simulink model "MBD_FOC_SENSORLESS_MODEL"  (R2022b)
settings: Solver=FixedStepDiscrete  StartTime=0.0  StopTime=9  FixedStep=.00005  RelTol=1e-3  EnableMultiTasking=on
PostLoadFcn:
  | MBD_FOC_SENSORLESS_DATA;
InitFcn:
  | MBD_FOC_SENSORLESS_DATA;
model workspace (MAT data in the model file):
  mwTaskManagerKernelLatency = 1e-06
values from neighbouring files (symbols this model uses):
  Iq_Ref_openLoop = 0.5    [MBD_FOC_SENSORLESS_DATA.m]
  PI_params = mcb.internal.SetControllerParameters(pmsm,inverter,PU_System,T_pwm,Ts,Ts_speed)    [MBD_FOC_SENSORLESS_DATA.m]
  PU_System = mcb_SetPUSystem(pmsm,inverter)    [MBD_FOC_SENSORLESS_DATA.m]
  PWM1max = 1600    [MBD_FOC_SENSORLESS_DATA.m]
  PWM_frequency = 20e3    (= 20000)    [MBD_FOC_SENSORLESS_DATA.m]
  Speed_Ref_openLoop = 500    [MBD_FOC_SENSORLESS_DATA.m]
  Ts = T_pwm    (= 5e-05)    [MBD_FOC_SENSORLESS_DATA.m]
  Ts_speed = 30*Ts    (= 0.0015)    [MBD_FOC_SENSORLESS_DATA.m]
undefined symbols (not defined in the file or in its folder): DiscIntNeverNeededParam, inverter, pmsm
libraries: mcbcontrolslib x9, simulink x4, slpidlib x3, mcbplantlib x1, autolibpmsmexterior x1
(part 1 of 2)
settings Model: Creator=M91449  LastModifiedBy=Administrator
settings SolverCC: AlgebraicLoopSolver=TrustRegion  PositivePriorityOrder=on  AutoInsertRateTranBlk=on  InsertRTBMode=Always
settings DataIOCC: LimitDataPoints=on  ReturnWorkspaceOutputs=off
settings OptimizationCC: DefaultParameterBehavior=Inlined  PassReuseOutputArgsAs=Individual arguments  ZeroExternalMemoryAtStartup=off  ZeroInternalMemoryAtStartup=off  MaxStackSize=64  OptimizationLevel=level1  OptimizationCustomize=off  EfficientTunableParamExpr=on
settings DebuggingCC: MultiTaskDSMMsg=none  ParameterOverflowMsg=none  ParameterTunabilityLossMsg=error  UnconnectedInputMsg=warning  UnconnectedOutputMsg=warning  UnconnectedLineMsg=warning  SFUnexpectedBacktrackingDiag=warning  SFNoUnconditionalDefaultTransitionDiag=warning  SFExecutionAtInitializationDiag=none  SFMachineParentedDataDiag=warning  ArithmeticOperatorsInVariantConditions=warning
settings HardwareCC: ProdBitPerPointer=32  ProdBitPerSizeT=32  ProdBitPerPtrDiffT=32  ProdLargestAtomicInteger=Long  ProdLargestAtomicFloat=Double  ProdWordSize=32  ProdHWDeviceType=ARM Compatible->ARM Cortex-M  HardwareBoardFeatureSet=SoCBlockset
settings ModelReferenceCC: EnableRefExpFcnMdlSchedulingChecks=on  ModelReferenceNumInstancesAllowed=Single  PropagateSignalLabelsOutOfModel=off
settings SFSimCC: SimUseLocalCustomCode=off  MATLABDynamicMemAlloc=off  CustomCodeUndefinedFunction=UseInterfaceOnly
settings RTWCC: Description=Embedded Coder  SystemTargetFile=ert.tlc  GenCodeOnly=on  TemplateMakefile=ert_default_tmf  GenerateReport=on  RTWUseLocalCustomCode=off  IncludeHyperlinkInReport=on  LaunchReport=on  GenerateCodeMetricsReport=on  DLArmComputeVersion=19.05
settings CodeAppCC: ForceParamTrailComments=on  IgnoreCustomStorageClasses=off  MaxIdLength=255  OperatorAnnotations=on  SimulinkDataObjDesc=on  SFDataObjDesc=on  InsertBlockDesc=on
settings ERTTargetCC: GenerateSampleERTMain=on  InlinedParameterPlacement=NonHierarchical  ERTCustomFileTemplate=example_file_process.tlc
settings ConfigComp: CovMetricSettings=dw  CovSaveCumulativeToWorkspaceVar=on  CovSaveSingleToWorkspaceVar=on  CovExternalEMLEnable=off

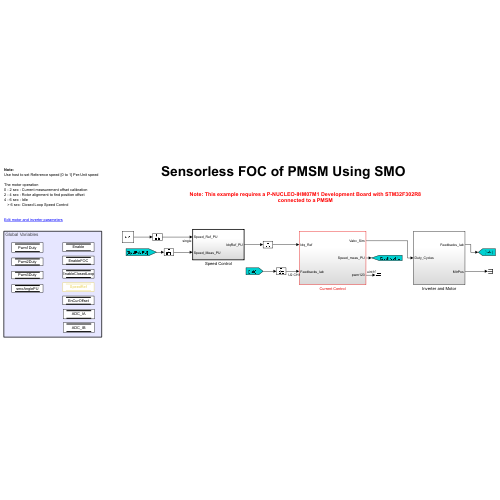
[thumbnail: Simulink's stored preview of the top-level diagram]
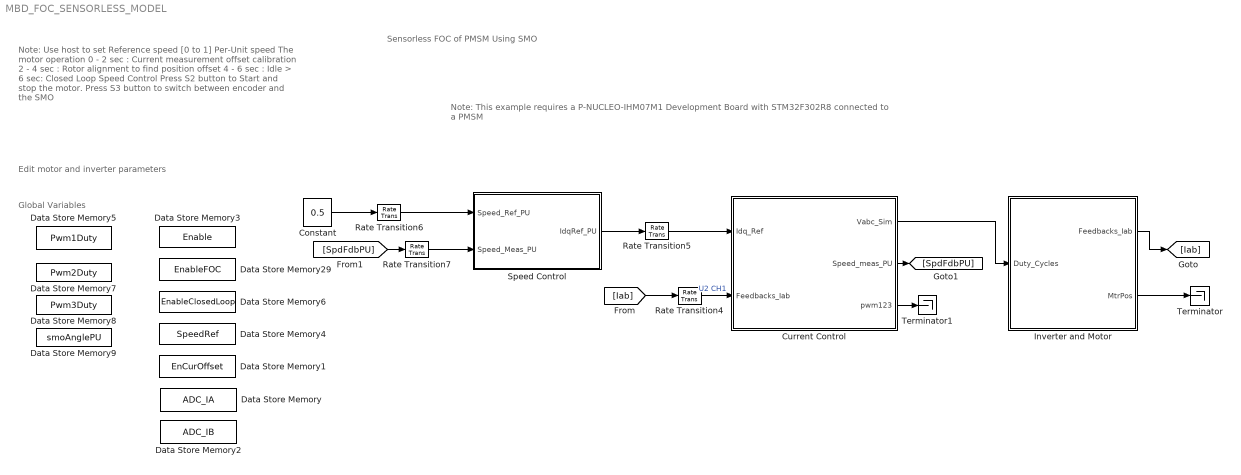
== system MBD_FOC_SENSORLESS_MODEL ==
  note: Edit motor and inverter parameters
  note: Note:
      | Use host to set Reference speed [0 to 1] Per-Unit speed
      |
      | The motor operation
      | 0 - 2 sec : Current measurement offset calibration
      | 2 - 4 sec : Rotor alignment to find position offset
      | 4 - 6 sec : Idle
      | > 6 sec: Closed Loop Speed Control
      |
      | Press S2 button to Start and stop the motor.
      | Press S3 button to switch between encoder and the SMO
  note: Global Variables
  note: Sensorless FOC of PMSM Using SMO
  note: Note: This example requires a P-NUCLEO-IHM07M1 Development Board with STM32F302R8 connected to a PMSM
  Constant : Constant  Value=0.5  OutDataTypeStr=single
  Current Control : Subsystem  VariantControl=Optimized
  Data Store Memory : DataStoreMemory  DataStoreName=ADC_IA  WriteAfterWriteMsg=warning  ShowAdditionalParam=off  OutDataTypeStr=uint16
  Data Store Memory1 : DataStoreMemory  DataStoreName=EnCurOffset  ShowAdditionalParam=off  OutDataTypeStr=boolean
  Data Store Memory2 : DataStoreMemory  DataStoreName=ADC_IB  WriteAfterWriteMsg=warning  ShowAdditionalParam=off  OutDataTypeStr=uint16
  Data Store Memory29 : DataStoreMemory  DataStoreName=EnableFOC  ShowAdditionalParam=off  OutDataTypeStr=boolean
  Data Store Memory3 : DataStoreMemory  DataStoreName=Enable  ShowAdditionalParam=off  OutDataTypeStr=boolean
  Data Store Memory4 : DataStoreMemory  DataStoreName=SpeedRef  ShowAdditionalParam=off  OutDataTypeStr=dataType
  Data Store Memory5 : DataStoreMemory  DataStoreName=Pwm1Duty  WriteAfterWriteMsg=warning  ShowAdditionalParam=off  OutDataTypeStr=uint16
  Data Store Memory6 : DataStoreMemory  DataStoreName=EnableClosedLoop  ShowAdditionalParam=off  OutDataTypeStr=boolean
  Data Store Memory7 : DataStoreMemory  DataStoreName=Pwm2Duty  WriteAfterWriteMsg=warning  ShowAdditionalParam=off  OutDataTypeStr=uint16
  Data Store Memory8 : DataStoreMemory  DataStoreName=Pwm3Duty  WriteAfterWriteMsg=warning  ShowAdditionalParam=off  OutDataTypeStr=uint16
  Data Store Memory9 : DataStoreMemory  DataStoreName=smoAnglePU  WriteAfterWriteMsg=warning  ShowAdditionalParam=off  OutDataTypeStr=dataType
  Inverter and Motor : Subsystem
  Rate Transition{4..7} (4 alike) : RateTransition  Deterministic=off
  Speed Control : Subsystem  TreatAsAtomicUnit=on  SystemSampleTime=Ts_speed
  Terminator : Terminator
  Terminator1 : Terminator
  wires:
  Current Control/1(Vabc_Sim) -> Inverter and Motor/1(Duty_Cycles)
  Rate Transition4/1 -> Current Control/2(Feedbacks_Iab)  "U2 CH1"
  Rate Transition6/1 -> Speed Control/1(Speed_Ref_PU)
  Rate Transition7/1 -> Speed Control/2(Speed_Meas_PU)
  Speed Control/1(IdqRef_PU) -> Rate Transition5/1
  Inverter and Motor/1(Feedbacks_Iab) -> [Iab]
  [Iab] -> Rate Transition4/1
  Rate Transition5/1 -> Current Control/1(Idq_Ref)
  Constant/1 -> Rate Transition6/1
  Inverter and Motor/2(MtrPos) -> Terminator/1
  Current Control/3(pwm123) -> Terminator1/1
  [SpdFdbPU] -> Rate Transition7/1
  Current Control/2(Speed_meas_PU) -> [SpdFdbPU]

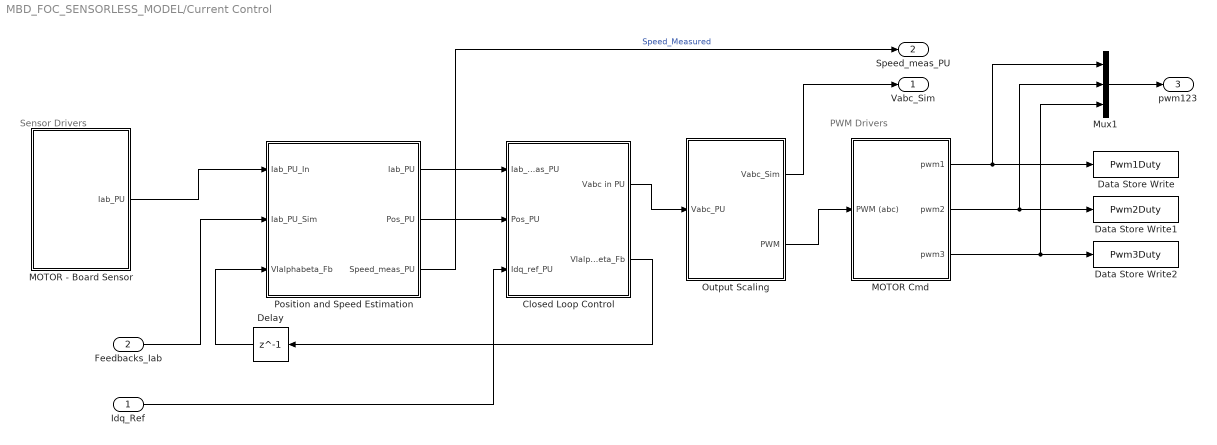
== system MBD_FOC_SENSORLESS_MODEL/Current Control ==
  note: Sensor Drivers
  note: PWM Drivers
  Idq_Ref : Inport
  Feedbacks_Iab : Inport  Port=2
  Closed Loop Control : Subsystem
  Data Store Write : DataStoreWrite  DataStoreName=Pwm1Duty  DataStoreElements=Pwm1Duty  IndexOptions=Index vector (dialog)  Indices=1  OutputSizes=1
  Data Store Write1 : DataStoreWrite  DataStoreName=Pwm2Duty  DataStoreElements=Pwm2Duty  IndexOptions=Index vector (dialog)  Indices=1  OutputSizes=1
  Data Store Write2 : DataStoreWrite  DataStoreName=Pwm3Duty  DataStoreElements=Pwm3Duty  IndexOptions=Index vector (dialog)  Indices=1  OutputSizes=1
  Delay : Delay  DelayLength=1
  MOTOR Cmd : Subsystem
  MOTOR - Board Sensor : Subsystem
  Mux1 : Mux  Inputs=3
  Output Scaling : Subsystem
  Position and Speed Estimation : Subsystem
  Vabc_Sim : Outport
  Speed_meas_PU : Outport  Port=2
  pwm123 : Outport  Port=3  OutDataTypeStr=uint16
  wires:
  Closed Loop Control/1(Vabc in PU) -> Output Scaling/1(Vabc_PU)
  Output Scaling/2(PWM) -> MOTOR Cmd/1(PWM (abc))
  Output Scaling/1(Vabc_Sim) -> Vabc_Sim/1
  Feedbacks_Iab/1 -> Position and Speed Estimation/2(Iab_PU_Sim)
  Position and Speed Estimation/1(Iab_PU) -> Closed Loop Control/1(Iab_meas_PU)
  Position and Speed Estimation/2(Pos_PU) -> Closed Loop Control/2(Pos_PU)
  MOTOR - Board Sensor/1(Iab_PU) -> Position and Speed Estimation/1(Iab_PU_In)
  Idq_Ref/1 -> Closed Loop Control/3(Idq_ref_PU)
  Closed Loop Control/2(VIalphabeta_Fb) -> Delay/1
  Delay/1 -> Position and Speed Estimation/3(VIalphabeta_Fb)
  Position and Speed Estimation/3(Speed_meas_PU) -> Speed_meas_PU/1  "Speed_Measured"
  MOTOR Cmd/3(pwm3) -> Mux1/3, Data Store Write2/1
  MOTOR Cmd/1(pwm1) -> Mux1/1, Data Store Write/1
  MOTOR Cmd/2(pwm2) -> Mux1/2, Data Store Write1/1
  Mux1/1 -> pwm123/1

== system MBD_FOC_SENSORLESS_MODEL/Inverter and Motor ==
  Duty_Cycles : Inport
  Codegeneration : Subsystem
  Simulation : Subsystem
  Variant Sink : VariantSink
  Variant Source : VariantSource
  Feedbacks_Iab : Outport  VectorParamsAs1DForOutWhenUnconnected=off
  MtrPos : Outport  Port=2
  wires:
  Codegeneration/1(Feedbacks_Iab) -> Variant Source/1
  Variant Sink/1 -> Codegeneration/1(Duty_Cycles)
  Simulation/1(Feedbacks_Iab) -> Variant Source/2
  Variant Sink/2 -> Simulation/1(Duty_Cycles)
  Variant Source/1 -> Feedbacks_Iab/1
  Duty_Cycles/1 -> Variant Sink/1
  Simulation/2(MtrPos) -> MtrPos/1

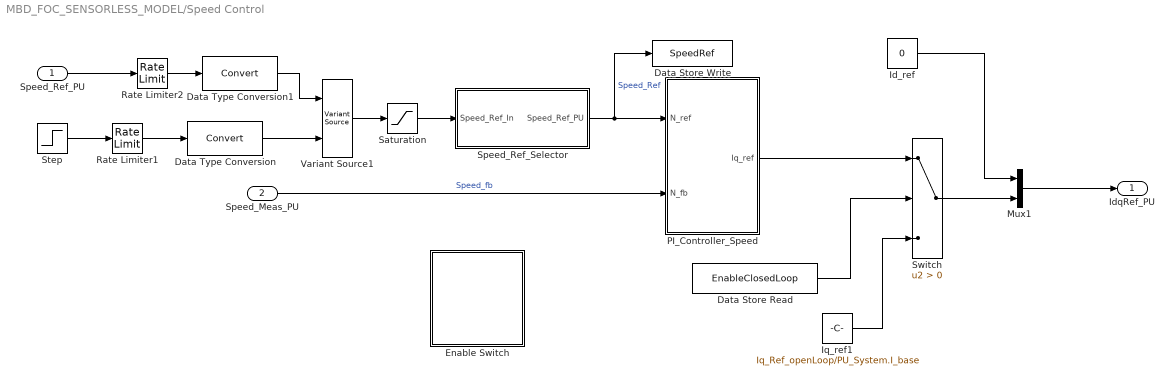
== system MBD_FOC_SENSORLESS_MODEL/Speed Control ==
  Speed_Ref_PU : Inport  OutDataTypeStr=single
  Speed_Meas_PU : Inport  Port=2
  Data Store Read : DataStoreRead  DataStoreName=EnableClosedLoop  IndexOptions=Index vector (dialog)  Indices=1  OutputSizes=1
  Data Store Write : DataStoreWrite  DataStoreName=SpeedRef  IndexOptions=Index vector (dialog)  Indices=1  OutputSizes=1
  Data Type Conversion : DataTypeConversion  SaturateOnIntegerOverflow=off  RndMeth=Floor
  Data Type Conversion1 : DataTypeConversion  SaturateOnIntegerOverflow=off  RndMeth=Floor
  Enable Switch : Subsystem  Variant=on  VariantControlMode=sim codegen switching
  Id_ref : Constant  Value=0  OutDataTypeStr=dataType  SampleTime=Ts_speed
  Iq_ref1 : Constant  Value=Iq_Ref_openLoop/PU_System.I_base  OutDataTypeStr=dataType  SampleTime=Ts_speed
  Mux1 : Mux  Inputs=2
  PI_Controller_Speed : Subsystem
  Rate Limiter1 : RateLimiter  RisingSlewLimit=0.5  FallingSlewLimit=-0.2  SampleTimeMode=inherited
  Rate Limiter2 : RateLimiter  RisingSlewLimit=0.5  FallingSlewLimit=-0.2  SampleTimeMode=inherited
  Saturation : Saturate  UpperLimit=(pmsm.N_max/PU_System.N_base)  LowerLimit=Speed_Ref_openLoop/PU_System.N_base
  Speed_Ref_Selector : Subsystem
  Step : Step  Time=5.5  Before=Speed_Ref_openLoop/PU_System.N_base  After=1.31  OutDataTypeStr=single
  Switch : Switch  Criteria=u2 > Threshold  SaturateOnIntegerOverflow=off  InputSameDT=off
  Variant Source1 : VariantSource
  IdqRef_PU : Outport  VectorParamsAs1DForOutWhenUnconnected=off
  wires:
  Speed_Meas_PU/1 -> PI_Controller_Speed/2(N_fb)  "Speed_fb"
  Id_ref/1 -> Mux1/1
  Mux1/1 -> IdqRef_PU/1
  Speed_Ref_Selector/1(Speed_Ref_PU) -> Data Store Write/1, PI_Controller_Speed/1(N_ref)  "Speed_Ref"
  Data Type Conversion/1 -> Variant Source1/2
  Step/1 -> Rate Limiter1/1
  Rate Limiter1/1 -> Data Type Conversion/1
  PI_Controller_Speed/1(Iq_ref) -> Switch/1
  Switch/1 -> Mux1/2
  Iq_ref1/1 -> Switch/3
  Data Store Read/1 -> Switch/2
  Variant Source1/1 -> Saturation/1
  Saturation/1 -> Speed_Ref_Selector/1(Speed_Ref_In)
  Speed_Ref_PU/1 -> Rate Limiter2/1
  Data Type Conversion1/1 -> Variant Source1/1
  Rate Limiter2/1 -> Data Type Conversion1/1

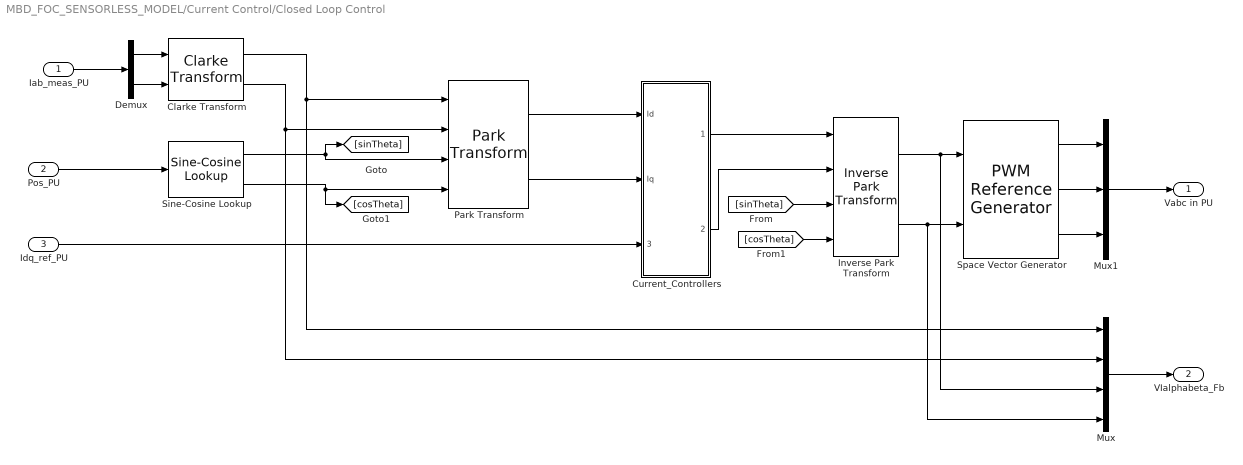
== system MBD_FOC_SENSORLESS_MODEL/Current Control/Closed Loop Control ==
  Iab_meas_PU : Inport
  Pos_PU : Inport  Port=2
  Idq_ref_PU : Inport  Port=3
  Clarke Transform : mcbcontrolslib/Clarke Transform  VariantControl=Variant2
  Current_Controllers : Subsystem
  Demux : Demux  Outputs=2
  Inverse Park Transform : mcbcontrolslib/Inverse Park Transform  AxisAlignment=D-axis
  Mux : Mux
  Mux1 : Mux  Inputs=3
  Park Transform : mcbcontrolslib/Park Transform  AxisAlignment=D-axis
  Sine-Cosine Lookup : mcbcontrolslib/Sine-Cosine Lookup  AngleInput=Per-unit  N_points=1024
  Space Vector Generator : mcbcontrolslib/PWM Reference Generator  inSignal=Valphabeta  modType=SVM: space vector modulation
  Vabc in PU : Outport  VectorParamsAs1DForOutWhenUnconnected=off
  VIalphabeta_Fb : Outport  Port=2
  wires:
  Current_Controllers/1(Vd_ref) -> Inverse Park Transform/1
  Inverse Park Transform/1 -> Mux/3, Space Vector Generator/1
  Park Transform/1 -> Current_Controllers/1(Id)
  Clarke Transform/1 -> Mux/1, Park Transform/1
  [sinTheta] -> Inverse Park Transform/3
  Sine-Cosine Lookup/1 -> Park Transform/3, [sinTheta]
  Clarke Transform/2 -> Mux/2, Park Transform/2
  Space Vector Generator/1 -> Mux1/1
  Space Vector Generator/3 -> Mux1/3
  Sine-Cosine Lookup/2 -> [cosTheta], Park Transform/4
  Space Vector Generator/2 -> Mux1/2
  Idq_ref_PU/1 -> Current_Controllers/3(Idq_ref_PU)
  Iab_meas_PU/1 -> Demux/1
  Inverse Park Transform/2 -> Mux/4, Space Vector Generator/2
  Demux/1 -> Clarke Transform/1
  Demux/2 -> Clarke Transform/2
  Park Transform/2 -> Current_Controllers/2(Iq)
  [cosTheta] -> Inverse Park Transform/4
  Current_Controllers/2(Vq_ref) -> Inverse Park Transform/2
  Mux1/1 -> Vabc in PU/1
  Pos_PU/1 -> Sine-Cosine Lookup/1
  Mux/1 -> VIalphabeta_Fb/1

== system MBD_FOC_SENSORLESS_MODEL/Current Control/MOTOR Cmd ==
  PWM (abc) : Inport
  Dead time Compensation : Bias  Bias=round( (inverter.deadtime/5e-5) *PWM1max )  SaturateOnIntegerOverflow=off
  Demux : Demux  Outputs=3
  Saturation low side turn on : Saturate  UpperLimit=PWM1max  LowerLimit=round( (inverter.deadtime/5e-5) *PWM1max )* 2
  int to uint : DataTypeConversion  OutDataTypeStr=uint16  ConvertRealWorld=Stored Integer (SI)  SaturateOnIntegerOverflow=off  RndMeth=Floor
  pwm1 : Outport  OutDataTypeStr=uint16
  pwm2 : Outport  Port=2  OutDataTypeStr=uint16
  pwm3 : Outport  Port=3  OutDataTypeStr=uint16
  wires:
  int to uint/1 -> Saturation low side turn on/1
  Dead time Compensation/1 -> int to uint/1
  PWM (abc)/1 -> Dead time Compensation/1
  Saturation low side turn on/1 -> Demux/1
  Demux/1 -> pwm1/1
  Demux/2 -> pwm2/1
  Demux/3 -> pwm3/1

== system MBD_FOC_SENSORLESS_MODEL/Current Control/MOTOR - Board Sensor ==
  Add2 : Sum  Inputs=+-  OutDataTypeStr=int16  RndMeth=Simplest
  Data Store Read : DataStoreRead  DataStoreName=EnCurOffset  IndexOptions=Index vector (dialog)  Indices=1  OutputSizes=1
  Data Store Read1 : DataStoreRead  DataStoreName=ADC_IA  IndexOptions=Index vector (dialog)  Indices=1  OutputSizes=1
  Data Store Read2 : DataStoreRead  DataStoreName=ADC_IB  IndexOptions=Index vector (dialog)  Indices=1  OutputSizes=1
  Mux2 : Mux  Inputs=2
  Offset1 : Subsystem
  Scale Ia Ib to (A) : DataTypeConversion  OutDataTypeStr=fixdt(1,16, 1.65/2048 / (inverter.Rshunt * inverter.opamp_Gain),0)  ConvertRealWorld=Stored Integer (SI)  SaturateOnIntegerOverflow=off  RndMeth=Floor
  To Per-Unit : Gain  Gain=inverter.invertingAmp/PU_System.I_base  OutMin=-1  OutMax=1  OutDataTypeStr=dataType  RndMeth=Zero
  Iab_PU : Outport  OutDataTypeStr=dataType  VectorParamsAs1DForOutWhenUnconnected=off
  wires:
  Mux2/1 -> Add2/1, Offset1/1(Iab)
  Scale Ia Ib to (A)/1 -> To Per-Unit/1  "Ia Ib"
  Offset1/1(Offset) -> Add2/2
  Add2/1 -> Scale Ia Ib to (A)/1
  Data Store Read/1 -> Offset1/Enable
  To Per-Unit/1 -> Iab_PU/1
  Data Store Read1/1 -> Mux2/1
  Data Store Read2/1 -> Mux2/2

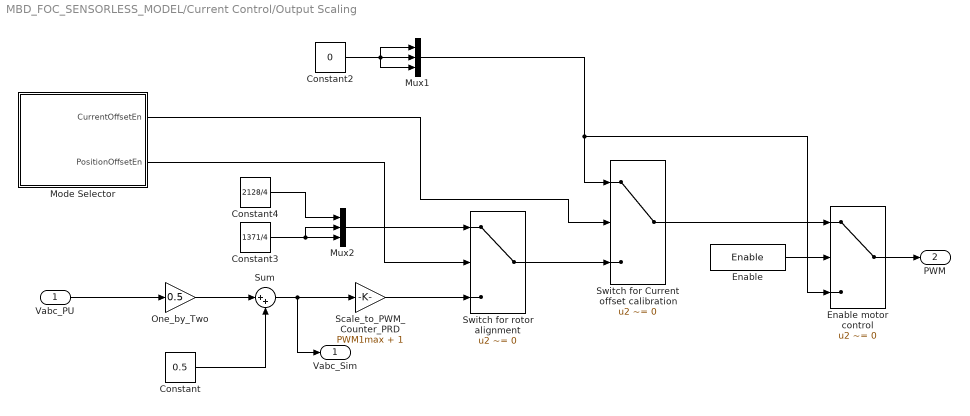
== system MBD_FOC_SENSORLESS_MODEL/Current Control/Output Scaling ==
  Vabc_PU : Inport
  Constant : Constant  Value=0.5  OutDataTypeStr=dataType  SampleTime=-1
  Constant2 : Constant  Value=0  OutDataTypeStr=Inherit: Inherit via back propagation
  Constant3 : Constant  Value=1371/4  OutDataTypeStr=Inherit: Inherit via back propagation
  Constant4 : Constant  Value=2128/4  OutDataTypeStr=Inherit: Inherit via back propagation
  Enable : DataStoreRead  DataStoreName=Enable  IndexOptions=Index vector (dialog)  Indices=1  OutputSizes=1
  Enable motor control : Switch  Criteria=u2 ~= 0  Threshold=250  SaturateOnIntegerOverflow=off  InputSameDT=off
  Mode Selector : Subsystem
  Mux1 : Mux  Inputs=3
  Mux2 : Mux  Inputs=3
  One_by_Two : Gain  Gain=0.5  RndMeth=Simplest  OutDataTypeStr=Inherit: Same as input
  Scale_to_PWM_Counter_PRD : Gain  Gain=PWM1max + 1  OutDataTypeStr=uint16  RndMeth=Simplest
  Sum : Sum  Inputs=|++
  Switch for Current offset calibration : Switch  Criteria=u2 ~= 0  Threshold=250  SaturateOnIntegerOverflow=off  InputSameDT=off
  Switch for rotor alignment : Switch  Criteria=u2 ~= 0  Threshold=250  SaturateOnIntegerOverflow=off  InputSameDT=off
  Vabc_Sim : Outport
  PWM : Outport  Port=2
  wires:
  Sum/1 -> Scale_to_PWM_Counter_PRD/1, Vabc_Sim/1
  Constant/1 -> Sum/2
  One_by_Two/1 -> Sum/1
  Switch for rotor alignment/1 -> Switch for Current offset calibration/3
  Vabc_PU/1 -> One_by_Two/1
  Mux2/1 -> Switch for rotor alignment/1
  Mux1/1 -> Switch for Current offset calibration/1, Enable motor control/3
  Constant2/1 -> Mux1/1, Mux1/3, Mux1/2
  Constant3/1 -> Mux2/3, Mux2/2
  Constant4/1 -> Mux2/1
  Enable/1 -> Enable motor control/2
  Mode Selector/2(PositionOffsetEn) -> Switch for rotor alignment/2
  Scale_to_PWM_Counter_PRD/1 -> Switch for rotor alignment/3
  Mode Selector/1(CurrentOffsetEn) -> Switch for Current offset calibration/2
  Enable motor control/1 -> PWM/1
  Switch for Current offset calibration/1 -> Enable motor control/1

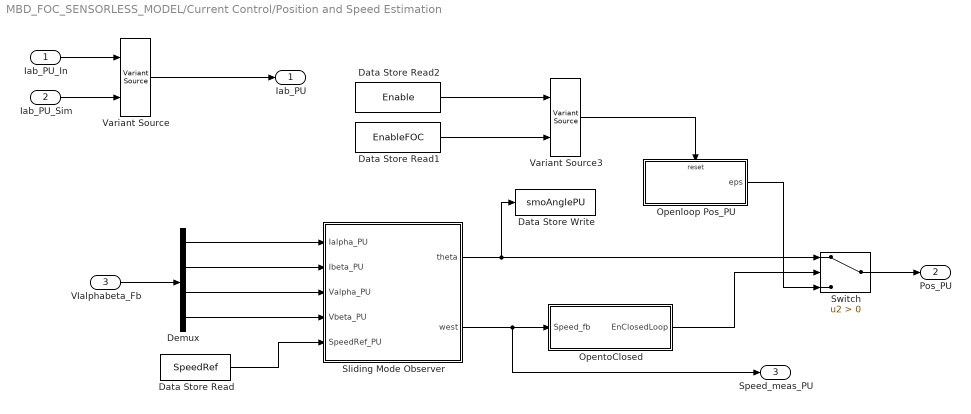
== system MBD_FOC_SENSORLESS_MODEL/Current Control/Position and Speed Estimation ==
  Iab_PU_In : Inport
  Iab_PU_Sim : Inport  Port=2
  VIalphabeta_Fb : Inport  Port=3
  Data Store Read : DataStoreRead  DataStoreName=SpeedRef  IndexOptions=Index vector (dialog)  Indices=1  OutputSizes=1
  Data Store Read1 : DataStoreRead  DataStoreName=EnableFOC  IndexOptions=Index vector (dialog)  Indices=1  OutputSizes=1
  Data Store Read2 : DataStoreRead  DataStoreName=Enable  IndexOptions=Index vector (dialog)  Indices=1  OutputSizes=1
  Data Store Write : DataStoreWrite  DataStoreName=smoAnglePU  IndexOptions=Index vector (dialog)  Indices=1  OutputSizes=1
  Demux : Demux
  Openloop Pos_PU : Subsystem  TreatAsAtomicUnit=on
  OpentoClosed : Subsystem
  Sliding Mode Observer : Subsystem
  Switch : Switch  Criteria=u2 > Threshold  SaturateOnIntegerOverflow=off  InputSameDT=off
  Variant Source : VariantSource
  Variant Source3 : VariantSource
  Iab_PU : Outport
  Pos_PU : Outport  Port=2
  Speed_meas_PU : Outport  Port=3
  wires:
  Iab_PU_In/1 -> Variant Source/1
  Iab_PU_Sim/1 -> Variant Source/2
  Variant Source/1 -> Iab_PU/1
  Data Store Read1/1 -> Variant Source3/2
  Variant Source3/1 -> Openloop Pos_PU/Reset
  Data Store Read2/1 -> Variant Source3/1
  VIalphabeta_Fb/1 -> Demux/1
  Demux/4 -> Sliding Mode Observer/4(Vbeta_PU)
  Data Store Read/1 -> Sliding Mode Observer/5(SpeedRef_PU)
  Demux/2 -> Sliding Mode Observer/2(Ibeta_PU)
  Demux/1 -> Sliding Mode Observer/1(Ialpha_PU)
  Demux/3 -> Sliding Mode Observer/3(Valpha_PU)
  Sliding Mode Observer/2(west) -> Speed_meas_PU/1, OpentoClosed/1(Speed_fb)
  OpentoClosed/1(EnClosedLoop) -> Switch/2
  Sliding Mode Observer/1(theta) -> Data Store Write/1, Switch/1
  Switch/1 -> Pos_PU/1
  Openloop Pos_PU/1(eps) -> Switch/3

== system MBD_FOC_SENSORLESS_MODEL/Inverter and Motor/Codegeneration ==
  Duty_Cycles : Inport
  Ground : Ground
  Terminator : Terminator
  Feedbacks_Iab : Outport  VectorParamsAs1DForOutWhenUnconnected=off
  wires:
  Ground/1 -> Feedbacks_Iab/1
  Duty_Cycles/1 -> Terminator/1

== system MBD_FOC_SENSORLESS_MODEL/Inverter and Motor/Simulation ==
  Duty_Cycles : Inport
  Bus Selector : BusSelector  OutputSignals=MtrPos
  Inverter : Subsystem
  Load_Profile (Torque) : Subsystem
  Sensor_Measurements : Subsystem
  Surface Mount PMSM : autolibpmsmexterior/Surface Mount PMSM  port_config=Torque  sim_type=Discrete  Ts=Ts  P=pmsm.p  Rs=pmsm.Rs + inverter.R_board  Ldq_=pmsm.Ld  KConstText=Permanent flux linkage constant (lambda_pm):  lambda_pm=pmsm.FluxPM  Ke=159.9771  Kt=1.323  mechanical=[pmsm.J, pmsm.B, 0]  idq0=[0 0]  theta_init=0  omega_init=0  KConst=pmsm.FluxPM  lambda_pm_calc=pmsm.FluxPM  RefBlkName='autolibpmsmexterior/Surface Mount PMSM'  aMode=5  Ldq="[0.0002      0.0002]"
  Terminator : Terminator
  Feedbacks_Iab : Outport  VectorParamsAs1DForOutWhenUnconnected=off
  MtrPos : Outport  Port=2
  wires:
  Duty_Cycles/1 -> Inverter/1(Duty_abc)
  Surface Mount PMSM/2 -> Sensor_Measurements/1(PhaseCurr)  "Iabc"
  Sensor_Measurements/1(Iab_fb) -> Feedbacks_Iab/1
  Load_Profile (Torque)/1(Load_Trq) -> Surface Mount PMSM/1
  Inverter/1(Vabc) -> Surface Mount PMSM/2
  Surface Mount PMSM/3 -> Terminator/1
  Surface Mount PMSM/1 -> Bus Selector/1
  Bus Selector/1 -> MtrPos/1  "<MtrPos>"

== system MBD_FOC_SENSORLESS_MODEL/Speed Control/Enable Switch ==
  Codegen : Subsystem  VariantControl=(codegen)
  Sim : Subsystem  VariantControl=(sim)

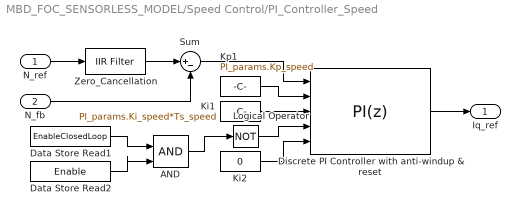
== system MBD_FOC_SENSORLESS_MODEL/Speed Control/PI_Controller_Speed ==
  N_ref : Inport
  N_fb : Inport  Port=2
  AND : Logic  IconShape=distinctive  AllPortsSameDT=off  OutDataTypeStr=boolean
  Data Store Read1 : DataStoreRead  DataStoreName=EnableClosedLoop  IndexOptions=Index vector (dialog)  Indices=1  OutputSizes=1
  Data Store Read2 : DataStoreRead  DataStoreName=Enable  IndexOptions=Index vector (dialog)  Indices=1  OutputSizes=1
  Discrete PI Controller with anti-windup & reset : slpidlib/PID Controller  Controller=PI  Form=Parallel  TimeDomain=Discrete-time  UseExternalTs=off  SampleTime=-1  IntegratorMethod=Forward Euler  FilterMethod=Forward Euler  ControllerParametersSource=external  P=1  I=1  UseKiTs=on  D=0  N=100  UseFilter=on  TunerSelectOption=Transfer Function Based (PID Tuner App)  InitialConditionSource=external  InitialConditionForIntegrator=0  InitialConditionForFilter=0  DifferentiatorICPrevScaledInput=0  ExternalReset=level  TrackingMode=off  Kt=1  LimitOutput=on  SatLimitsSource=internal  UpperSaturationLimit=1  LowerSaturationLimit=-1  LinearizeAsGain=on  AntiWindupMode=clamping  Kb=1  LimitIntegrator=off  UpperIntegratorSaturationLimit=inf  LowerIntegratorSaturationLimit=-inf  RndMeth=Simplest  POutMin=[]  POutMax=[]  IOutMin=[]  IOutMax=[]  DOutMin=[]  DOutMax=[]  NOutMin=[]  NOutMax=[]  SumOutMin=[]  SumOutMax=[]  SaturationOutDataTypeStr=Inherit: Inherit via back propagation  SaturationOutMin=[]  SaturationOutMax=[]  PParamMin=[]  PParamMax=[]  IParamMin=[]  IParamMax=[]  DParamMin=[]  DParamMax=[]  NParamMin=[]  NParamMax=[]  KbParamMin=[]  KbParamMax=[]  KtParamMin=[]  KtParamMax=[]  KbOutMin=[]  KbOutMax=[]  KtOutMin=[]  KtOutMax=[]  IntegratorOutMin=[]  IntegratorOutMax=[]  FilterOutMin=[]  FilterOutMax=[]  SumI1OutMin=[]  SumI1OutMax=[]  SumI2OutMin=[]  SumI2OutMax=[]  SumI3OutMin=[]  SumI3OutMax=[]  SumI4OutMin=[]  SumI4OutMax=[]  SumDOutMin=[]  SumDOutMax=[]  DifferentiatorOutMin=[]  DifferentiatorOutMax=[]  FilterDiffOutCoefMin=[]  FilterDiffOutCoefMax=[]  ReciprocalOutMin=[]  ReciprocalOutMax=[]  SumDenOutMin=[]  SumDenOutMax=[]  SumNumOutMin=[]  SumNumOutMax=[]  DivideOutMin=[]  DivideOutMax=[]  UdiffTsProdOutMin=[]  UdiffTsProdOutMax=[]  NTsProdOutMin=[]  NTsProdOutMax=[]  UintegralTsProdOutMin=[]  UintegralTsProdOutMax=[]  UngainTsProdOutMin=[]  UngainTsProdOutMax=[]  ClampingZeroOutDataTypeStr=Inherit: Inherit via back propagation  ClampingZeroOutMin=[]  ClampingZeroOutMax=[]  FilterDenConstantOutDataTypeStr=Inherit: Inherit via back propagation  FilterDenConstantOutMin=[]  FilterDenConstantOutMax=[]  PCopyOutDataTypeStr=Inherit: Inherit via back propagation  PCopyOutMin=[]  PCopyOutMax=[]  NCopyOutDataTypeStr=Inherit: Inherit via back propagation  NCopyOutMin=[]  NCopyOutMax=[]  IntegratorContinuousStateAttributes=''  IntegratorStateMustResolveToSignalObject=off  IntegratorRTWStateStorageClass=Auto  FilterContinuousStateAttributes=''  FilterStateMustResolveToSignalObject=off  FilterRTWStateStorageClass=Auto  ParallelPVariant=ExternalParameters  IdealPVariant=Disabled  IVariant=ExternalParameters  DVariant=Disabled  IntegratorVariant=Discrete  SatVariant=Enabled  AWVariant=DiscClampingParallel  PCopyVariant=Disabled  TRVariant=Disabled  FdbkBlocksVariant=Forward  IdealPFdbkVariant=Disabled  SatFdbkVariant=Disabled  DerivativeFilterVariant=Disabled  NVariant=Disabled  NCopyVariant=Disabled_SignalSpec  FilterICVariant=Disabled  IntegratorICVariant=ExternalICs  ExternalResetVariant=ExternalReset  TRSumVariant=Passthrough  SumFdbkVariant=Disabled  SumVariant=Sum_PI  TsampFilterVariant=InternalTs  TsampNgainVariant=Passthrough  TsampIntegralVariant=Passthrough  ExternalSaturationOutDataTypeStr=Inherit: Same as second input
  Ki1 : Constant  Value=PI_params.Ki_speed*Ts_speed  OutDataTypeStr=dataType  SampleTime=-1
  Ki2 : Constant  Value=0  OutDataTypeStr=dataType  SampleTime=-1
  Kp1 : Constant  Value=PI_params.Kp_speed  OutDataTypeStr=dataType  SampleTime=-1
  Logical Operator : Logic  Operator=NOT  IconShape=distinctive  AllPortsSameDT=off  OutDataTypeStr=boolean
  Sum : Sum  Inputs=|+-  OutDataTypeStr=Inherit: Same as first input
  Zero_Cancellation : mcbcontrolslib/IIR Filter  VariantControl=Low Pass Filter  VariantSelect=Low-pass  Filter_constant=0.001*(Ts_speed/Ts)  advancedSettings=off  Ts=50e-6  cutOff_freq=98.4464
  Iq_ref : Outport  VectorParamsAs1DForOutWhenUnconnected=off
  wires:
  Discrete PI Controller with anti-windup & reset/1 -> Iq_ref/1
  Ki1/1 -> Discrete PI Controller with anti-windup & reset/3
  Kp1/1 -> Discrete PI Controller with anti-windup & reset/2
  N_fb/1 -> Sum/2
  N_ref/1 -> Zero_Cancellation/1
  Sum/1 -> Discrete PI Controller with anti-windup & reset/1
  Logical Operator/1 -> Discrete PI Controller with anti-windup & reset/4
  Ki2/1 -> Discrete PI Controller with anti-windup & reset/5
  Zero_Cancellation/1 -> Sum/1
  AND/1 -> Logical Operator/1
  Data Store Read1/1 -> AND/1
  Data Store Read2/1 -> AND/2

== system MBD_FOC_SENSORLESS_MODEL/Speed Control/Speed_Ref_Selector ==
  Speed_Ref_In : Inport
  Constant : Constant  Value=0  OutDataTypeStr=dataType
  Data Store Read1 : DataStoreRead  DataStoreName=EnableFOC  IndexOptions=Index vector (dialog)  Indices=1  OutputSizes=1
  Switch : Switch  Criteria=u2 > Threshold  Threshold=0.5  SaturateOnIntegerOverflow=off  InputSameDT=off
  Speed_Ref_PU : Outport
  wires:
  Switch/1 -> Speed_Ref_PU/1
  Constant/1 -> Switch/3
  Speed_Ref_In/1 -> Switch/1
  Data Store Read1/1 -> Switch/2

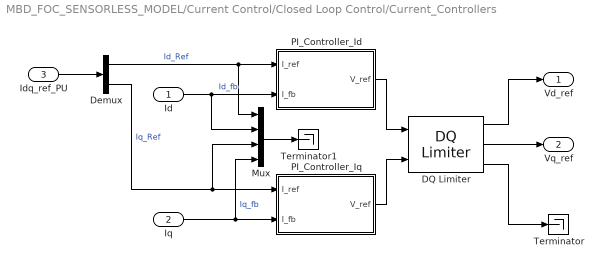
== system MBD_FOC_SENSORLESS_MODEL/Current Control/Closed Loop Control/Current_Controllers ==
  Id : Inport
  Iq : Inport  Port=2
  Idq_ref_PU : Inport  Port=3
  DQ Limiter : mcbcontrolslib/DQ Limiter  satMethodInputType=Specify via dialog  satMethodSelected=D-Q equivalence  satLimitInputType=Specify via dialog  Vmax=0.95
  Demux : Demux  Outputs=2
  Mux : Mux
  PI_Controller_Id : Subsystem
  PI_Controller_Iq : Subsystem
  Terminator : Terminator
  Terminator1 : Terminator
  Vd_ref : Outport  VectorParamsAs1DForOutWhenUnconnected=off
  Vq_ref : Outport  Port=2  VectorParamsAs1DForOutWhenUnconnected=off
  wires:
  Iq/1 -> Mux/4, PI_Controller_Iq/2(I_fb)  "Iq_fb"
  Id/1 -> Mux/2, PI_Controller_Id/2(I_fb)  "Id_fb"
  Demux/1 -> Mux/1, PI_Controller_Id/1(I_ref)  "Id_Ref"
  Demux/2 -> Mux/3, PI_Controller_Iq/1(I_ref)  "Iq_Ref"
  Idq_ref_PU/1 -> Demux/1
  PI_Controller_Id/1(V_ref) -> DQ Limiter/1
  PI_Controller_Iq/1(V_ref) -> DQ Limiter/2
  DQ Limiter/1 -> Vd_ref/1
  DQ Limiter/2 -> Vq_ref/1
  DQ Limiter/3 -> Terminator/1
  Mux/1 -> Terminator1/1

== system MBD_FOC_SENSORLESS_MODEL/Current Control/MOTOR - Board Sensor/Offset1 ==
  Iab : Inport
  Enable : EnablePort
  Offset : Outport
  wires:
  Iab/1 -> Offset/1

== system MBD_FOC_SENSORLESS_MODEL/Current Control/Output Scaling/Mode Selector ==
  Delay : Delay  DelayLength=1
  NOT : Logic  Operator=NOT  IconShape=distinctive  AllPortsSameDT=off  OutDataTypeStr=boolean
  Subsystem1 : Subsystem
  Up Counter : Subsystem
  CurrentOffsetEn : Outport
  PositionOffsetEn : Outport  Port=2
  wires:
  Subsystem1/2(PositionOffset) -> PositionOffsetEn/1
  Up Counter/1(Count) -> Subsystem1/1(Count)
  Subsystem1/1(Current Offset) -> CurrentOffsetEn/1
  Delay/1 -> NOT/1
  NOT/1 -> Up Counter/Enable
  Subsystem1/3(EnableFOC) -> Delay/1

== system MBD_FOC_SENSORLESS_MODEL/Current Control/Position and Speed Estimation/Openloop Pos_PU ==
  Reset : ResetPort  DisableCoverage=on
  Constant : Constant  Value=Speed_Ref_openLoop/PU_System.N_base  OutDataTypeStr=dataType
  Data Type Conversion : DataTypeConversion  OutDataTypeStr=fixdt(1,32,20)  ConvertRealWorld=Stored Integer (SI)  SaturateOnIntegerOverflow=off  RndMeth=Floor
  Discrete-Time Integrator : DiscreteIntegrator  IntegratorMethod=Accumulation: Forward Euler  gainval=0.002  SampleTime=Ts  OutDataTypeStr=fixdt(1,32,20)  LimitOutput=on  UpperSaturationLimit=500/PU_System.N_base  LowerSaturationLimit=0  ICPrevOutput=DiscIntNeverNeededParam  ICPrevScaledInput=DiscIntNeverNeededParam
  Gain : Gain  Gain=Ts*PU_System.N_base*pmsm.p/60  OutDataTypeStr=dataType  ParamDataTypeStr=Inherit: Same as input
  Position Generator : mcbcontrolslib/Position Generator  AngleOutput=Per-unit  ThetaSource=External  ThetaInput=5e-4  DataType=double  ExternalReset=none  Offset=0
  eps : Outport
  wires:
  Constant/1 -> Data Type Conversion/1
  Data Type Conversion/1 -> Discrete-Time Integrator/1
  Discrete-Time Integrator/1 -> Gain/1
  Position Generator/1 -> eps/1
  Gain/1 -> Position Generator/1

== system MBD_FOC_SENSORLESS_MODEL/Current Control/Position and Speed Estimation/OpentoClosed ==
  Speed_fb : Inport
  Chart : Stateflow chart  TreatAsAtomicUnit=on
  Data Store Read5 : DataStoreRead  DataStoreName=Enable  IndexOptions=Index vector (dialog)  Indices=1  OutputSizes=1
  Data Store Write2 : DataStoreWrite  DataStoreName=EnableClosedLoop  IndexOptions=Index vector (dialog)  Indices=1  OutputSizes=1
  Data Type Conversion : DataTypeConversion  OutDataTypeStr=boolean  RndMeth=Simplest  SaturateOnIntegerOverflow=off
  Enable Closed Loop : Constant  OutDataTypeStr=uint16
  Enable Closed Loop1 : Constant  Value=Speed_Ref_openLoop/PU_System.N_base  OutDataTypeStr=dataType
  Open Loop Start-up : Constant  Value=0  OutDataTypeStr=uint16
  Switch2 : Switch  Criteria=u2 > Threshold  Threshold=1  SaturateOnIntegerOverflow=off  InputSameDT=off
  Terminator : Terminator
  EnClosedLoop : Outport
  wires:
  Open Loop Start-up/1 -> Switch2/3
  Data Store Read5/1 -> Chart/3(En)
  Chart/1(Mode) -> Switch2/2
  Switch2/1 -> Data Type Conversion/1
  Speed_fb/1 -> Chart/2(SpeedFb)
  Enable Closed Loop/1 -> Switch2/1
  Enable Closed Loop1/1 -> Chart/1(Limit)
  Chart/2(SpeedCtrl) -> Terminator/1
  Data Type Conversion/1 -> EnClosedLoop/1, Data Store Write2/1

== system MBD_FOC_SENSORLESS_MODEL/Current Control/Position and Speed Estimation/Sliding Mode Observer ==
  Ialpha_PU : Inport
  Ibeta_PU : Inport  Port=2
  Valpha_PU : Inport  Port=3
  Vbeta_PU : Inport  Port=4
  SpeedRef_PU : Inport  Port=5
  SMO Implemetation : Subsystem
  Scaling : Subsystem
  theta : Outport
  west : Outport  Port=2
  wires:
  Scaling/1(Ialpha) -> SMO Implemetation/1(ialfa)
  Ialpha_PU/1 -> Scaling/1(Ialpha_PU)
  Scaling/2(Ibeta) -> SMO Implemetation/2(ibeta)
  Scaling/3(Valpha) -> SMO Implemetation/3(valfa)
  Scaling/4(Vbeta) -> SMO Implemetation/4(vbeta)
  Scaling/5(SpeedRef) -> SMO Implemetation/5(wref)
  Vbeta_PU/1 -> Scaling/4(Vbeta_PU)
  Valpha_PU/1 -> Scaling/3(Valpha_PU)
  Ibeta_PU/1 -> Scaling/2(Ibeta_PU)
  SpeedRef_PU/1 -> Scaling/5(SpeedRef_PU)
  SMO Implemetation/1(theta) -> theta/1
  SMO Implemetation/2(west) -> west/1

== system MBD_FOC_SENSORLESS_MODEL/Inverter and Motor/Simulation/Inverter ==
  Duty_abc : Inport
  Average-Value Inverter : mcbplantlib/Average-Value Inverter
  Constant2 : Constant  Value=inverter.V_dc  OutDataTypeStr=single  SampleTime=-1
  Data Type Conversion1 : DataTypeConversion  OutDataTypeStr=single  RndMeth=Simplest  SaturateOnIntegerOverflow=off
  Vabc : Outport  VectorParamsAs1DForOutWhenUnconnected=off
  wires:
  Average-Value Inverter/1 -> Vabc/1
  Data Type Conversion1/1 -> Average-Value Inverter/1
  Duty_abc/1 -> Data Type Conversion1/1
  Constant2/1 -> Average-Value Inverter/2

== system MBD_FOC_SENSORLESS_MODEL/Inverter and Motor/Simulation/Load_Profile (Torque) ==
  Data Type Conversion : DataTypeConversion  OutDataTypeStr=single  SaturateOnIntegerOverflow=off  RndMeth=Floor
  IIR Filter : mcbcontrolslib/IIR Filter  VariantControl=Low Pass Filter  VariantSelect=Low-pass  Filter_constant=0.01  advancedSettings=off  Ts=50e-6  cutOff_freq=32.1525
  Rate Limiter1 : RateLimiter  RisingSlewLimit=0.5  FallingSlewLimit=-0.2  SampleTimeMode=inherited
  Step : Step  Commented=on  Time=5  Before=0.0* pmsm.T_rated  After=0.25* pmsm.T_rated
  Step1 : Step  Commented=on  Time=8  Before=0.25* pmsm.T_rated  After=pmsm.T_rated
  Step2 : Step  Commented=on  Time=8  Before=1  After=0
  Switch : Switch  Criteria=u2 > Threshold  SaturateOnIntegerOverflow=off  InputSameDT=off
  Load_Trq : Outport  VectorParamsAs1DForOutWhenUnconnected=off
  wires:
  IIR Filter/1 -> Load_Trq/1
  Data Type Conversion/1 -> IIR Filter/1
  Switch/1 -> Rate Limiter1/1
  Step1/1 -> Switch/3
  Step/1 -> Switch/1
  Step2/1 -> Switch/2
  Rate Limiter1/1 -> Data Type Conversion/1

== system MBD_FOC_SENSORLESS_MODEL/Inverter and Motor/Simulation/Sensor_Measurements ==
  PhaseCurr : Inport
  Data Type Conversion4 : DataTypeConversion  OutDataTypeStr=single  RndMeth=Simplest  SaturateOnIntegerOverflow=off
  Delay1 : Delay  DelayLength=PI_params.delay_Currents
  Inverting OpAmp : Gain  Gain=1/PU_System.I_base  OutDataTypeStr=dataType  RndMeth=Simplest
  Selector : Selector  InputPortWidth=3  IndexOptions=Index vector (dialog)  Indices=[1 2]  OutputSizes=1
  Iab_fb : Outport  VectorParamsAs1DForOutWhenUnconnected=off
  wires:
  Selector/1 -> Inverting OpAmp/1
  PhaseCurr/1 -> Data Type Conversion4/1
  Data Type Conversion4/1 -> Delay1/1
  Delay1/1 -> Selector/1  "Iab_fb"
  Inverting OpAmp/1 -> Iab_fb/1

== system MBD_FOC_SENSORLESS_MODEL/Speed Control/Enable Switch/Codegen ==
  note: Toggle between enable and disable on press on Button S2
  Constant : Constant  OutDataTypeStr=boolean
  Triggered Subsystem : Subsystem  TreatAsAtomicUnit=on
  wires:
  Constant/1 -> Triggered Subsystem/Trigger

== system MBD_FOC_SENSORLESS_MODEL/Speed Control/Enable Switch/Sim ==
  Constant : Constant  OutDataTypeStr=Inherit: Inherit via back propagation
  Data Store Write : DataStoreWrite  DataStoreName=Enable  IndexOptions=Index vector (dialog)  Indices=1  OutputSizes=1
  wires:
  Constant/1 -> Data Store Write/1

== system MBD_FOC_SENSORLESS_MODEL/Current Control/Closed Loop Control/Current_Controllers/PI_Controller_Id ==
  I_ref : Inport
  I_fb : Inport  Port=2
  AND : Logic  IconShape=distinctive  AllPortsSameDT=off  OutDataTypeStr=boolean
  Data Store Read : DataStoreRead  DataStoreName=Enable  IndexOptions=Index vector (dialog)  Indices=1  OutputSizes=1
  Data Store Read1 : DataStoreRead  DataStoreName=EnableFOC  IndexOptions=Index vector (dialog)  Indices=1  OutputSizes=1
  Discrete PI Controller with anti-windup & reset : slpidlib/PID Controller  Controller=PI  Form=Parallel  TimeDomain=Discrete-time  UseExternalTs=off  SampleTime=-1  IntegratorMethod=Forward Euler  FilterMethod=Forward Euler  ControllerParametersSource=external  P=1  I=1  UseKiTs=on  D=0  N=100  UseFilter=on  TunerSelectOption=Transfer Function Based (PID Tuner App)  InitialConditionSource=external  InitialConditionForIntegrator=0  InitialConditionForFilter=0  DifferentiatorICPrevScaledInput=0  ExternalReset=level  TrackingMode=off  Kt=1  LimitOutput=on  SatLimitsSource=internal  UpperSaturationLimit=1  LowerSaturationLimit=-1  LinearizeAsGain=on  AntiWindupMode=clamping  Kb=1  LimitIntegrator=off  UpperIntegratorSaturationLimit=inf  LowerIntegratorSaturationLimit=-inf  RndMeth=Simplest  POutMin=[]  POutMax=[]  IOutMin=[]  IOutMax=[]  DOutMin=[]  DOutMax=[]  NOutMin=[]  NOutMax=[]  SumOutMin=[]  SumOutMax=[]  SaturationOutDataTypeStr=Inherit: Inherit via back propagation  SaturationOutMin=[]  SaturationOutMax=[]  PParamMin=[]  PParamMax=[]  IParamMin=[]  IParamMax=[]  DParamMin=[]  DParamMax=[]  NParamMin=[]  NParamMax=[]  KbParamMin=[]  KbParamMax=[]  KtParamMin=[]  KtParamMax=[]  KbOutMin=[]  KbOutMax=[]  KtOutMin=[]  KtOutMax=[]  IntegratorOutMin=[]  IntegratorOutMax=[]  FilterOutMin=[]  FilterOutMax=[]  SumI1OutMin=[]  SumI1OutMax=[]  SumI2OutMin=[]  SumI2OutMax=[]  SumI3OutMin=[]  SumI3OutMax=[]  SumI4OutMin=[]  SumI4OutMax=[]  SumDOutMin=[]  SumDOutMax=[]  DifferentiatorOutMin=[]  DifferentiatorOutMax=[]  FilterDiffOutCoefMin=[]  FilterDiffOutCoefMax=[]  ReciprocalOutMin=[]  ReciprocalOutMax=[]  SumDenOutMin=[]  SumDenOutMax=[]  SumNumOutMin=[]  SumNumOutMax=[]  DivideOutMin=[]  DivideOutMax=[]  UdiffTsProdOutMin=[]  UdiffTsProdOutMax=[]  NTsProdOutMin=[]  NTsProdOutMax=[]  UintegralTsProdOutMin=[]  UintegralTsProdOutMax=[]  UngainTsProdOutMin=[]  UngainTsProdOutMax=[]  ClampingZeroOutDataTypeStr=Inherit: Inherit via back propagation  ClampingZeroOutMin=[]  ClampingZeroOutMax=[]  FilterDenConstantOutDataTypeStr=Inherit: Inherit via back propagation  FilterDenConstantOutMin=[]  FilterDenConstantOutMax=[]  PCopyOutDataTypeStr=Inherit: Inherit via back propagation  PCopyOutMin=[]  PCopyOutMax=[]  NCopyOutDataTypeStr=Inherit: Inherit via back propagation  NCopyOutMin=[]  NCopyOutMax=[]  IntegratorContinuousStateAttributes=''  IntegratorStateMustResolveToSignalObject=off  IntegratorRTWStateStorageClass=Auto  FilterContinuousStateAttributes=''  FilterStateMustResolveToSignalObject=off  FilterRTWStateStorageClass=Auto  ParallelPVariant=ExternalParameters  IdealPVariant=Disabled  IVariant=ExternalParameters  DVariant=Disabled  IntegratorVariant=Discrete  SatVariant=Enabled  AWVariant=DiscClampingParallel  PCopyVariant=Disabled  TRVariant=Disabled  FdbkBlocksVariant=Forward  IdealPFdbkVariant=Disabled  SatFdbkVariant=Disabled  DerivativeFilterVariant=Disabled  NVariant=Disabled  NCopyVariant=Disabled_SignalSpec  FilterICVariant=Disabled  IntegratorICVariant=ExternalICs  ExternalResetVariant=ExternalReset  TRSumVariant=Passthrough  SumFdbkVariant=Disabled  SumVariant=Sum_PI  TsampFilterVariant=InternalTs  TsampNgainVariant=Passthrough  TsampIntegralVariant=Passthrough  ExternalSaturationOutDataTypeStr=Inherit: Same as second input
  Ki : Constant  Value=PI_params.Ki_i*Ts/2  OutDataTypeStr=dataType  SampleTime=-1
  Ki1 : Constant  Value=0  OutDataTypeStr=dataType  SampleTime=-1
  Kp : Constant  Value=PI_params.Kp_i/2  OutDataTypeStr=dataType2  SampleTime=-1
  Logical Operator : Logic  Operator=NOT  IconShape=distinctive  AllPortsSameDT=off  OutDataTypeStr=boolean
  Sum : Sum  Inputs=|+-  OutDataTypeStr=Inherit: Same as first input
  V_ref : Outport  VectorParamsAs1DForOutWhenUnconnected=off
  wires:
  I_ref/1 -> Sum/1
  I_fb/1 -> Sum/2
  Data Store Read1/1 -> AND/1
  Discrete PI Controller with anti-windup & reset/1 -> V_ref/1
  Sum/1 -> Discrete PI Controller with anti-windup & reset/1
  Kp/1 -> Discrete PI Controller with anti-windup & reset/2
  Ki/1 -> Discrete PI Controller with anti-windup & reset/3
  Logical Operator/1 -> Discrete PI Controller with anti-windup & reset/4
  Ki1/1 -> Discrete PI Controller with anti-windup & reset/5
  Data Store Read/1 -> AND/2
  AND/1 -> Logical Operator/1

== system MBD_FOC_SENSORLESS_MODEL/Current Control/Closed Loop Control/Current_Controllers/PI_Controller_Iq ==
  I_ref : Inport
  I_fb : Inport  Port=2
  AND : Logic  IconShape=distinctive  AllPortsSameDT=off  OutDataTypeStr=boolean
  Data Store Read : DataStoreRead  DataStoreName=Enable  IndexOptions=Index vector (dialog)  Indices=1  OutputSizes=1
  Data Store Read1 : DataStoreRead  DataStoreName=EnableFOC  IndexOptions=Index vector (dialog)  Indices=1  OutputSizes=1
  Discrete PI Controller with anti-windup & reset : slpidlib/PID Controller  Controller=PI  Form=Parallel  TimeDomain=Discrete-time  UseExternalTs=off  SampleTime=-1  IntegratorMethod=Forward Euler  FilterMethod=Forward Euler  ControllerParametersSource=external  P=1  I=1  UseKiTs=on  D=0  N=100  UseFilter=on  TunerSelectOption=Transfer Function Based (PID Tuner App)  InitialConditionSource=external  InitialConditionForIntegrator=0  InitialConditionForFilter=0  DifferentiatorICPrevScaledInput=0  ExternalReset=level  TrackingMode=off  Kt=1  LimitOutput=on  SatLimitsSource=internal  UpperSaturationLimit=1  LowerSaturationLimit=-1  LinearizeAsGain=on  AntiWindupMode=clamping  Kb=1  LimitIntegrator=off  UpperIntegratorSaturationLimit=inf  LowerIntegratorSaturationLimit=-inf  RndMeth=Simplest  POutMin=[]  POutMax=[]  IOutMin=[]  IOutMax=[]  DOutMin=[]  DOutMax=[]  NOutMin=[]  NOutMax=[]  SumOutMin=[]  SumOutMax=[]  SaturationOutDataTypeStr=Inherit: Inherit via back propagation  SaturationOutMin=[]  SaturationOutMax=[]  PParamMin=[]  PParamMax=[]  IParamMin=[]  IParamMax=[]  DParamMin=[]  DParamMax=[]  NParamMin=[]  NParamMax=[]  KbParamMin=[]  KbParamMax=[]  KtParamMin=[]  KtParamMax=[]  KbOutMin=[]  KbOutMax=[]  KtOutMin=[]  KtOutMax=[]  IntegratorOutMin=[]  IntegratorOutMax=[]  FilterOutMin=[]  FilterOutMax=[]  SumI1OutMin=[]  SumI1OutMax=[]  SumI2OutMin=[]  SumI2OutMax=[]  SumI3OutMin=[]  SumI3OutMax=[]  SumI4OutMin=[]  SumI4OutMax=[]  SumDOutMin=[]  SumDOutMax=[]  DifferentiatorOutMin=[]  DifferentiatorOutMax=[]  FilterDiffOutCoefMin=[]  FilterDiffOutCoefMax=[]  ReciprocalOutMin=[]  ReciprocalOutMax=[]  SumDenOutMin=[]  SumDenOutMax=[]  SumNumOutMin=[]  SumNumOutMax=[]  DivideOutMin=[]  DivideOutMax=[]  UdiffTsProdOutMin=[]  UdiffTsProdOutMax=[]  NTsProdOutMin=[]  NTsProdOutMax=[]  UintegralTsProdOutMin=[]  UintegralTsProdOutMax=[]  UngainTsProdOutMin=[]  UngainTsProdOutMax=[]  ClampingZeroOutDataTypeStr=Inherit: Inherit via back propagation  ClampingZeroOutMin=[]  ClampingZeroOutMax=[]  FilterDenConstantOutDataTypeStr=Inherit: Inherit via back propagation  FilterDenConstantOutMin=[]  FilterDenConstantOutMax=[]  PCopyOutDataTypeStr=Inherit: Inherit via back propagation  PCopyOutMin=[]  PCopyOutMax=[]  NCopyOutDataTypeStr=Inherit: Inherit via back propagation  NCopyOutMin=[]  NCopyOutMax=[]  IntegratorContinuousStateAttributes=''  IntegratorStateMustResolveToSignalObject=off  IntegratorRTWStateStorageClass=Auto  FilterContinuousStateAttributes=''  FilterStateMustResolveToSignalObject=off  FilterRTWStateStorageClass=Auto  ParallelPVariant=ExternalParameters  IdealPVariant=Disabled  IVariant=ExternalParameters  DVariant=Disabled  IntegratorVariant=Discrete  SatVariant=Enabled  AWVariant=DiscClampingParallel  PCopyVariant=Disabled  TRVariant=Disabled  FdbkBlocksVariant=Forward  IdealPFdbkVariant=Disabled  SatFdbkVariant=Disabled  DerivativeFilterVariant=Disabled  NVariant=Disabled  NCopyVariant=Disabled_SignalSpec  FilterICVariant=Disabled  IntegratorICVariant=ExternalICs  ExternalResetVariant=ExternalReset  TRSumVariant=Passthrough  SumFdbkVariant=Disabled  SumVariant=Sum_PI  TsampFilterVariant=InternalTs  TsampNgainVariant=Passthrough  TsampIntegralVariant=Passthrough  ExternalSaturationOutDataTypeStr=Inherit: Same as second input
  Ki : Constant  Value=PI_params.Ki_i*Ts/2  OutDataTypeStr=dataType  SampleTime=-1
  Kp : Constant  Value=PI_params.Kp_i/2  OutDataTypeStr=dataType2  SampleTime=-1
  Kp1 : Constant  Value=0  OutDataTypeStr=dataType  SampleTime=-1
  Logical Operator : Logic  Operator=NOT  IconShape=distinctive  AllPortsSameDT=off  OutDataTypeStr=boolean
  Sum : Sum  Inputs=|+-  OutDataTypeStr=Inherit: Same as first input
  V_ref : Outport  VectorParamsAs1DForOutWhenUnconnected=off
  wires:
  Discrete PI Controller with anti-windup & reset/1 -> V_ref/1
  Data Store Read1/1 -> AND/1
  I_fb/1 -> Sum/2
  I_ref/1 -> Sum/1
  Kp/1 -> Discrete PI Controller with anti-windup & reset/2
  Sum/1 -> Discrete PI Controller with anti-windup & reset/1
  Ki/1 -> Discrete PI Controller with anti-windup & reset/3
  Logical Operator/1 -> Discrete PI Controller with anti-windup & reset/4
  Kp1/1 -> Discrete PI Controller with anti-windup & reset/5
  Data Store Read/1 -> AND/2
  AND/1 -> Logical Operator/1

== system MBD_FOC_SENSORLESS_MODEL/Current Control/Output Scaling/Mode Selector/Subsystem1 ==
  Count : Inport
  AND : Logic  IconShape=distinctive  AllPortsSameDT=off  OutDataTypeStr=boolean
  Compare To Constant : simulink/Logic and Bit Operations/Compare To Constant  relop=>=  const=2  OutDataTypeStr=boolean
  Compare To Constant1 : simulink/Logic and Bit Operations/Compare To Constant  relop=<  const=1  OutDataTypeStr=boolean
  Compare To Constant2 : simulink/Logic and Bit Operations/Compare To Constant  relop=<  const=2  OutDataTypeStr=boolean
  Compare To Constant3 : simulink/Logic and Bit Operations/Compare To Constant  relop=>  const=1  OutDataTypeStr=boolean
  Data Store Write : DataStoreWrite  DataStoreName=EnCurOffset  IndexOptions=Index vector (dialog)  Indices=1  OutputSizes=1
  Data Store Write1 : DataStoreWrite  DataStoreName=EnableFOC  IndexOptions=Index vector (dialog)  Indices=1  OutputSizes=1
  Gain : Gain  Gain=1/PWM_frequency  OutDataTypeStr=dataType2  RndMeth=Simplest
  Current Offset : Outport
  PositionOffset : Outport  Port=2
  EnableFOC : Outport  Port=3
  wires:
  Count/1 -> Gain/1
  Gain/1 -> Compare To Constant1/1, Compare To Constant3/1, Compare To Constant2/1, Compare To Constant/1
  Compare To Constant1/1 -> Data Store Write/1, Current Offset/1
  Compare To Constant2/1 -> AND/2
  Compare To Constant3/1 -> AND/1
  AND/1 -> PositionOffset/1
  Compare To Constant/1 -> Data Store Write1/1, EnableFOC/1

== system MBD_FOC_SENSORLESS_MODEL/Current Control/Output Scaling/Mode Selector/Up Counter ==
  Enable : EnablePort  StatesWhenEnabling=reset
  Add1 : Sum  SaturateOnIntegerOverflow=on
  Constant : Constant  OutDataTypeStr=uint32
  Delay : Delay  DelayLength=1
  Count : Outport  InitialOutput=0
  wires:
  Delay/1 -> Add1/2
  Add1/1 -> Count/1, Delay/1
  Constant/1 -> Add1/1

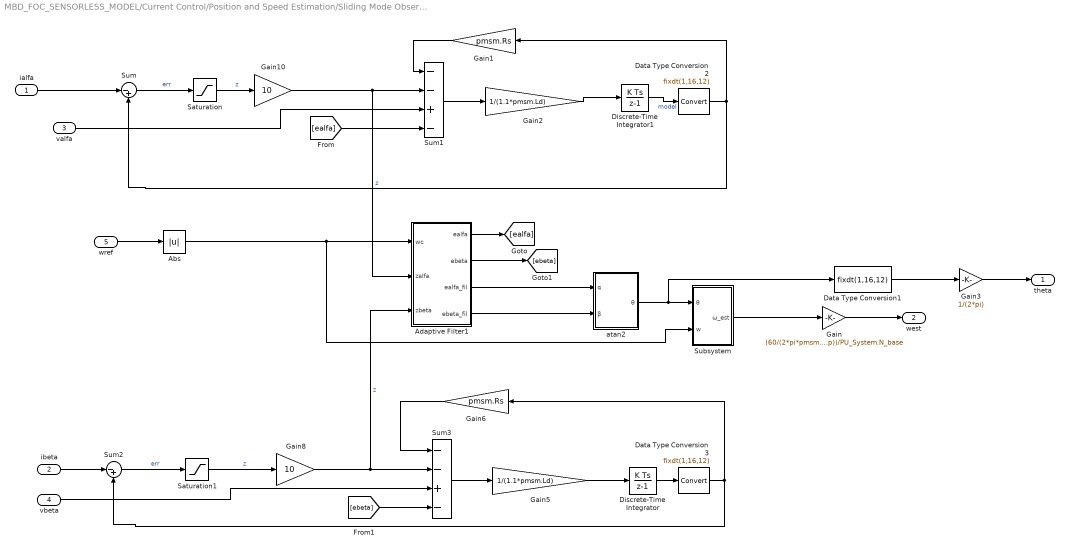
== system MBD_FOC_SENSORLESS_MODEL/Current Control/Position and Speed Estimation/Sliding Mode Observer/SMO Implemetation ==
  ialfa : Inport
  ibeta : Inport  Port=2
  valfa : Inport  Port=3
  vbeta : Inport  Port=4
  wref : Inport  Port=5
  Abs : Abs  SaturateOnIntegerOverflow=off
  Adaptive Filter1 : Subsystem
  Data Type Conversion1 : DataTypeConversion  OutDataTypeStr=fixdt(1,16,12)  SaturateOnIntegerOverflow=off  RndMeth=Floor
  Data Type Conversion2 : DataTypeConversion  OutDataTypeStr=fixdt(1,16,12)  SaturateOnIntegerOverflow=off  RndMeth=Floor
  Data Type Conversion3 : DataTypeConversion  OutDataTypeStr=fixdt(1,16,12)  SaturateOnIntegerOverflow=off  RndMeth=Floor
  Discrete-Time Integrator : DiscreteIntegrator  SampleTime=-1  OutDataTypeStr=fixdt(1,32,17)  ICPrevOutput=DiscIntNeverNeededParam  ICPrevScaledInput=DiscIntNeverNeededParam
  Discrete-Time Integrator1 : DiscreteIntegrator  SampleTime=-1  OutDataTypeStr=fixdt(1,32,17)  ICPrevOutput=DiscIntNeverNeededParam  ICPrevScaledInput=DiscIntNeverNeededParam
  Gain : Gain  Gain=(60/(2*pi*pmsm.p))/PU_System.N_base  OutDataTypeStr=dataType
  Gain1 : Gain  Gain=pmsm.Rs  OutDataTypeStr=fixdt(1,16,12)
  Gain10 : Gain  Gain=10  OutDataTypeStr=fixdt(1,16,8)
  Gain2 : Gain  Gain=1/(1.1*pmsm.Ld)  OutDataTypeStr=fixdt(1,32,14)
  Gain3 : Gain  Gain=1/(2*pi)  OutDataTypeStr=dataType
  Gain5 : Gain  Gain=1/(1.1*pmsm.Ld)  OutDataTypeStr=fixdt(1,32,14)
  Gain6 : Gain  Gain=pmsm.Rs  OutDataTypeStr=fixdt(1,16,12)
  Gain8 : Gain  Gain=10  OutDataTypeStr=fixdt(1,16,8)
  Saturation : Saturate  UpperLimit=0.7  LowerLimit=-0.7
  Saturation1 : Saturate  UpperLimit=0.7  LowerLimit=-0.7
  Subsystem : Subsystem
  Sum : Sum  Inputs=|-+  AccumDataTypeStr=fixdt(1,16,10)  OutDataTypeStr=fixdt(1,16,10)
  Sum1 : Sum  Inputs=--+-  AccumDataTypeStr=fixdt(1,16,8)  OutDataTypeStr=fixdt(1,16,8)
  Sum2 : Sum  Inputs=|-+  AccumDataTypeStr=fixdt(1,16,10)  OutDataTypeStr=fixdt(1,16,10)
  Sum3 : Sum  Inputs=--+-  AccumDataTypeStr=fixdt(1,16,8)  OutDataTypeStr=fixdt(1,16,8)
  atan2 : Subsystem
  theta : Outport  VectorParamsAs1DForOutWhenUnconnected=off
  west : Outport  Port=2  VectorParamsAs1DForOutWhenUnconnected=off
  wires:
  atan2/1(θ) -> Data Type Conversion1/1, Subsystem/1(θ)
  Discrete-Time Integrator1/1 -> Data Type Conversion2/1  "model"
  ialfa/1 -> Sum/1
  Sum/1 -> Saturation/1  "err"
  Sum1/1 -> Gain2/1
  Gain2/1 -> Discrete-Time Integrator1/1
  Saturation/1 -> Gain10/1  "z"
  Subsystem/1(ω_est) -> Gain/1
  Sum2/1 -> Saturation1/1  "err"
  ibeta/1 -> Sum2/1
  Sum3/1 -> Gain5/1
  Gain5/1 -> Discrete-Time Integrator/1
  Discrete-Time Integrator/1 -> Data Type Conversion3/1
  vbeta/1 -> Sum3/3
  Gain6/1 -> Sum3/1
  Gain1/1 -> Sum1/1
  valfa/1 -> Sum1/3
  wref/1 -> Abs/1
  Adaptive Filter1/1(ealfa) -> [ealfa]
  Adaptive Filter1/2(ebeta) -> [ebeta]
  Adaptive Filter1/3(ealfa_fil) -> atan2/1(α)
  Adaptive Filter1/4(ebeta_fil) -> atan2/2(β)
  Data Type Conversion1/1 -> Gain3/1
  Saturation1/1 -> Gain8/1  "z"
  Data Type Conversion2/1 -> Sum/2, Gain1/1
  Data Type Conversion3/1 -> Sum2/2, Gain6/1
  Gain10/1 -> Sum1/2, Adaptive Filter1/2(zalfa)  "z"
  Gain8/1 -> Adaptive Filter1/3(zbeta), Sum3/2  "z"
  Gain/1 -> west/1
  [ealfa] -> Sum1/4
  [ebeta] -> Sum3/4
  Gain3/1 -> theta/1
  Abs/1 -> Subsystem/2(w), Adaptive Filter1/1(wc)

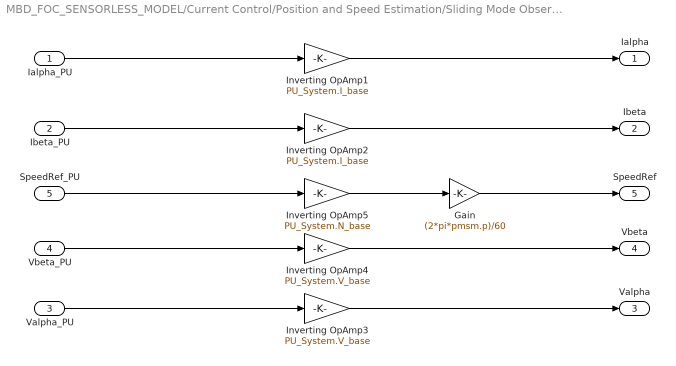
== system MBD_FOC_SENSORLESS_MODEL/Current Control/Position and Speed Estimation/Sliding Mode Observer/Scaling ==
  Ialpha_PU : Inport
  Ibeta_PU : Inport  Port=2
  Valpha_PU : Inport  Port=3
  Vbeta_PU : Inport  Port=4
  SpeedRef_PU : Inport  Port=5
  Gain : Gain  Gain=(2*pi*pmsm.p)/60  OutDataTypeStr=fixdt(1,16,3)
  Inverting OpAmp1 : Gain  Gain=PU_System.I_base  OutDataTypeStr=fixdt(1,16,12)  RndMeth=Simplest
  Inverting OpAmp2 : Gain  Gain=PU_System.I_base  OutDataTypeStr=fixdt(1,16,12)  RndMeth=Simplest
  Inverting OpAmp3 : Gain  Gain=PU_System.V_base  OutDataTypeStr=fixdt(1,16,11)  RndMeth=Simplest
  Inverting OpAmp4 : Gain  Gain=PU_System.V_base  OutDataTypeStr=fixdt(1,16,11)  RndMeth=Simplest
  Inverting OpAmp5 : Gain  Gain=PU_System.N_base  OutDataTypeStr=fixdt(1,16,2)  RndMeth=Simplest
  Ialpha : Outport
  Ibeta : Outport  Port=2
  Valpha : Outport  Port=3
  Vbeta : Outport  Port=4
  SpeedRef : Outport  Port=5
  wires:
  Vbeta_PU/1 -> Inverting OpAmp4/1
  SpeedRef_PU/1 -> Inverting OpAmp5/1
  Inverting OpAmp2/1 -> Ibeta/1
  Inverting OpAmp3/1 -> Valpha/1
  Ibeta_PU/1 -> Inverting OpAmp2/1
  Inverting OpAmp4/1 -> Vbeta/1
  Ialpha_PU/1 -> Inverting OpAmp1/1
  Inverting OpAmp1/1 -> Ialpha/1
  Valpha_PU/1 -> Inverting OpAmp3/1
  Inverting OpAmp5/1 -> Gain/1
  Gain/1 -> SpeedRef/1
